simulink model "fixedWing"  (R2024b)
settings: Solver=ode1  StartTime=0.0  StopTime=20  FixedStep=0.001  RelTol=1e-3
undefined symbols (not defined in the file): initial_fw_state, params
libraries: uavutilslib x1
settings Model: PacingRate=0.010000  Creator=William Riis  LastModifiedBy=William Riis
settings DataIOCC: SaveFormat=StructureWithTime  SaveState=on

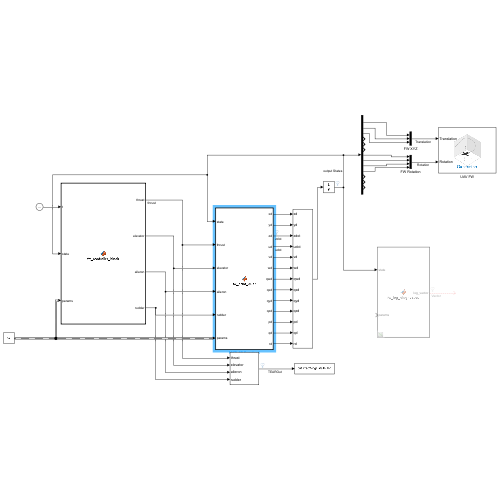
[thumbnail: Simulink's stored preview of the top-level diagram]
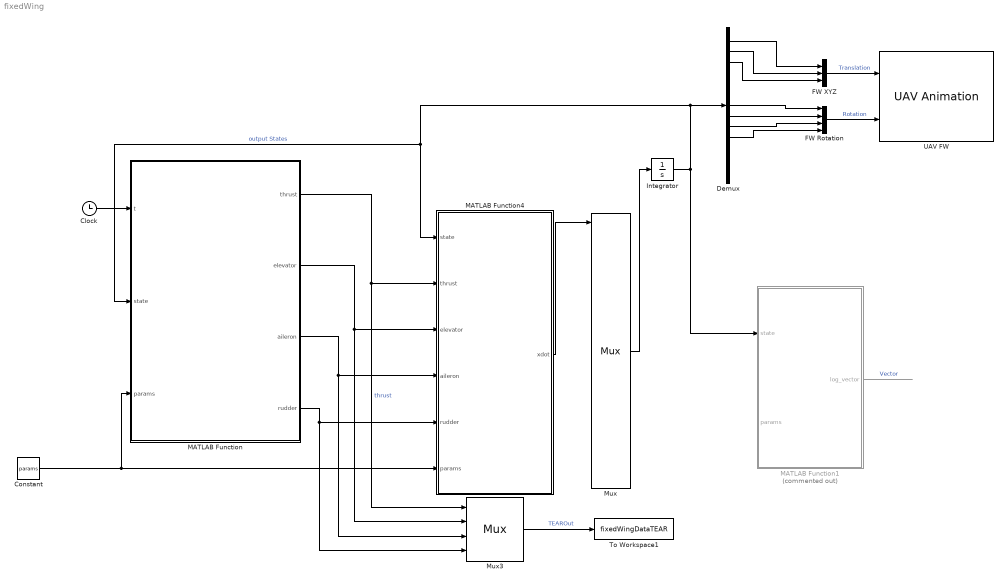
== system fixedWing ==
  Clock : Clock
  Constant : Constant  Value=params  OutDataTypeStr=Bus: paramsBus
  Demux : Demux  Outputs=13
  FW Rotation : Mux
  FW XYZ : Mux  Inputs=3
  Integrator : Integrator  InitialCondition=initial_fw_state
  MATLAB Function : MATLAB Function  TreatAsAtomicUnit=on
  MATLAB Function1 : MATLAB Function  Commented=on  TreatAsAtomicUnit=on
  MATLAB Function4 : MATLAB Function  TreatAsAtomicUnit=on
  Mux : Mux  Inputs=13
      settings: DisplayOption=signals
  Mux3 : Mux
      settings: DisplayOption=signals
  To Workspace1 : ToWorkspace  VariableName=fixedWingDataTEAR  SaveFormat=Structure With Time  SampleTime=-1
      settings: Save2DSignal=2-D array (concatenate along first dimension)
  UAV FW : uavutilslib/UAV Animation  NumUAV=1  DynamicUAVConfig=off  UAVType=FixedWing  UAVSize=20  UAVColor=[1 0 0]  UAVTrajectoryAlpha=1  InertialZDirection=Down  RotationFormat=Quaternion  DrawMarkers=off  SampleTime=.01
  wires:
  Integrator/1 -> MATLAB Function1/1(state), Demux/1, MATLAB Function4/1(state), MATLAB Function/2(state)  "output States"
  Mux3/1 -> To Workspace1/1  "TEAROut"
  FW XYZ/1 -> UAV FW/1  "Translation"
  MATLAB Function/4(rudder) -> Mux3/4, MATLAB Function4/5(rudder)
  MATLAB Function/3(aileron) -> Mux3/3, MATLAB Function4/4(aileron)
  MATLAB Function/2(elevator) -> Mux3/2, MATLAB Function4/3(elevator)
  MATLAB Function/1(thrust) -> Mux3/1, MATLAB Function4/2(thrust)  "thrust"
  FW Rotation/1 -> UAV FW/2  "Rotation"
  Mux/1 -> Integrator/1
  Clock/1 -> MATLAB Function/1(t)
  MATLAB Function1/1(log_vector) -> ?  "Vector"
  Demux/1 -> FW XYZ/1
  Demux/2 -> FW XYZ/2
  Demux/3 -> FW XYZ/3
  Demux/7 -> FW Rotation/1
  Demux/8 -> FW Rotation/2
  Demux/9 -> FW Rotation/3
  Demux/10 -> FW Rotation/4
  MATLAB Function4/1(xdot) -> Mux/1
  ? -> Mux/2
  ? -> Mux/3  "zdot"
  ? -> Mux/4  "udot"
  ? -> Mux/5
  ? -> Mux/6
  ? -> Mux/7
  ? -> Mux/8
  ? -> Mux/9
  ? -> Mux/10
  ? -> Mux/11
  ? -> Mux/12
  ? -> Mux/13
  Constant/1 -> MATLAB Function/3(params), MATLAB Function4/6(params)

== matlab function fixedWing/MATLAB Function1 ==
  data: state input; log_vector output; params input
function log_vector = fw_log_diagnostics(state, params)
% Logs diagnostics from aircraft state for debugging purposes

% === Unpack State ===
u = state(4); v = state(5); w = state(6);
phi = state(7); theta = state(8); psi = state(9);

% === Aircraft Constants (Fixed-Wing Specific with Prefixes) ===
rho = params.rho;
S   = params.fw_S;
CL0 = params.fw_CL0;
CL_alpha = params.fw_CL_alpha;
CD0 = params.fw_CD0;
k   = params.fw_k;

% === Velocity & Angles ===
V_b = [u; v; w];
V = norm(V_b) + 1e-3;
alpha = atan2(w, u);
qbar = 0.5 * rho * V^2;

% === Aero Coefficients & Forces ===
CL = CL0 + CL_alpha * alpha;
CD = CD0 + k * CL^2;
L = CL * qbar * S;
D = CD * qbar * S;

% === Direction Vectors ===
V_hat = V_b / V;
drag_dir = -V_hat;
lift_dir = cross([0; 1; 0], drag_dir);
lift_dir = lift_dir / max(1e-6, norm(lift_dir));

% === Logged Output Vector ===
% [V, alpha, CL, CD, L, D, V_hat(1:3), lift_dir(1:3)]
log_vector = [V; alpha; CL; CD; L; D; V_hat; lift_dir];
end

== matlab function fixedWing/MATLAB Function4 ==
  data: state input; thrust input; elevator input; aileron input; rudder input; xdot output; params input
function xdot = fw_6dof_quat(state, thrust, elevator, aileron, rudder, params)
% FW_6DOF_QUAT  Rigid-body 6-DoF fixed-wing with wind-axis aero
%
% State (13x1): [x y z u v w q0 q1 q2 q3 p q r]'
%   x,y,z   : position in NED (m)  (Z down)
%   u,v,w   : body translational velocities (m/s)  (inertial-relative)
%   q0..q3  : quaternion q_BN (N->Body), scalar-first (Hamilton)
%   p,q,r   : body rates (rad/s)
%
% Inputs:
%   thrust   : propulsive thrust along +x_B (N)
%   elevator : elevator deflection (rad)
%   aileron  : aileron deflection  (rad)
%   rudder   : rudder deflection   (rad)
%
% Params (required fields; uses safe defaults if missing):
%   rho,S,b,c,g, wind_ned(3x1)
%   Ix,Iy,Iz,Ixz (preferred) OR J (3x3)
%   Aero coeffs: CL0, CL_alpha, CL_q, CL_de,
%                CD0, k (=induced), CDa, CD_q, CD_de,
%                CY_beta, CY_p, CY_r, CY_da, CY_dr,
%                Cl_beta, Cl_p, Cl_r, Cl_da, Cl_dr,
%                Cm0, Cm_alpha, Cm_q, Cm_de,
%                Cn_beta, Cn_p, Cn_r, Cn_da, Cn_dr
%   r_T (3x1): thrust offset from CG in body (m), optional (default [0;0;0])

% -------- unpack state
x = state(1); y = state(2); z = state(3); %#ok<NASGU>
u = state(4); v = state(5); w = state(6);
qBN = state(7:10);
p = state(11); q = state(12); r = state(13);

% -------- params & defaults
rho  = getdef(params,'rho',1.225);
S    = getdef(params,'S',0.25);
b    = getdef(params,'b',1.2);
c    = getdef(params,'c',S/max(b,eps));
g    = getdef(params,'g',9.81);
wind = getdef(params,'wind_ned',[0;0;0]);

% Inertia (allow Ixz coupling)
if all(isfield(params, {'Ix','Iy','Iz'}))
    Ix  = params.Ix; Iy = params.Iy; Iz = params.Iz;
    Ixz = getdef(params,'Ixz',0);
    J   = [Ix, 0, -Ixz;
           0,  Iy, 0;
          -Ixz,0,  Iz];
else
    J = getdef(params,'J',diag([0.045 0.065 0.085]));
end

% Aero coefficients (provide zeros if missing)
CL0   = getdef(params,'CL0',0);
CL_a  = getdef(params,'CL_alpha',0);
CL_q  = getdef(params,'CL_q',0);
CL_de = getdef(params,'CL_de',0);

CD0   = getdef(params,'CD0',0.01);
k_ind = getdef(params,'k',0.03);
CD_a  = getdef(params,'CDa',0);
CD_q  = getdef(params,'CD_q',0);
CD_de = getdef(params,'CD_de',0);

CY_b  = getdef(params,'CY_beta',0);
CY_p  = getdef(params,'CY_p',0);
CY_r  = getdef(params,'CY_r',0);
CY_da = getdef(params,'CY_da',0);
CY_dr = getdef(params,'CY_dr',0);

Cl_b  = getdef(params,'Cl_beta',0);
Cl_p  = getdef(params,'Cl_p',0);
Cl_r  = getdef(params,'Cl_r',0);
Cl_da = getdef(params,'Cl_da',0);
Cl_dr = getdef(params,'Cl_dr',0);

Cm0   = getdef(params,'Cm0',0);
Cm_a  = getdef(params,'Cm_alpha',0);
Cm_q  = getdef(params,'Cm_q',0);
Cm_de = getdef(params,'Cm_de',0);

Cn_b  = getdef(params,'Cn_beta',0);
Cn_p  = getdef(params,'Cn_p',0);
Cn_r  = getdef(params,'Cn_r',0);
Cn_da = getdef(params,'Cn_da',0);
Cn_dr = getdef(params,'Cn_dr',0);

r_T = getdef(params,'r_T',[0;0;0]);

% -------- rotations
R_BN = quatNED_to_body(qBN);  % N->B
R_NB = R_BN.';                % B->N

% -------- kinematics: position time-derivative in NED
v_b   = [u; v; w];
v_ned = R_NB * v_b;
x_dot = v_ned(1);
y_dot = v_ned(2);
z_dot = v_ned(3);

% -------- air-relative velocity in body
v_air_b = v_b - R_BN*wind;    % (R_BN*wind) is wind expressed in body
ua = v_air_b(1); va = v_air_b(2); wa = v_air_b(3);
Va = max(1e-3, norm(v_air_b));

alpha = atan2(wa, ua);                     % angle of attack
beta  = asin( clamp(va/Va, -1, 1) );       % sideslip

qbar = 0.5 * rho * Va^2;
p_hat = (b/(2*Va)) * p;
q_hat = (c/(2*Va)) * q;
r_hat = (b/(2*Va)) * r;

% -------- aerodynamic coefficients
CL = CL0 + CL_a*alpha + CL_q*q_hat + CL_de*elevator;
CD = CD0 + k_ind*CL^2 + CD_a*alpha + CD_q*q_hat + CD_de*elevator;
CY = CY_b*beta + CY_p*p_hat + CY_r*r_hat + CY_da*aileron + CY_dr*rudder;

Cl = Cl_b*beta + Cl_p*p_hat + Cl_r*r_hat + Cl_da*aileron + Cl_dr*rudder;
Cm = Cm0 + Cm_a*alpha + Cm_q*q_hat + Cm_de*elevator;
Cn = Cn_b*beta + Cn_p*p_hat + Cn_r*r_hat + Cn_da*aileron + Cn_dr*rudder;

% -------- wind-axis → body conversion for forces
% In wind axes, F_w = [ -D,  Y,  -L ] * qbar*S
F_w = qbar*S * [-CD; CY; -CL];

% Rotation from body->wind (C_b^w), then use its transpose for wind->body
ca = cos(alpha); sa = sin(alpha);
cb = cos(beta);  sb = sin(beta);
C_b_w = [  ca*cb,  sb,    sa*cb;
          -ca*sb,  cb,   -sa*sb;
          -sa,     0,      ca  ];
R_wb = C_b_w.';               % wind -> body
F_aero_b = R_wb * F_w;

% -------- aerodynamic moments in body
M_aero_b = qbar*S * [ b*Cl; c*Cm; b*Cn ];

% -------- thrust force & moment
F_thrust_b = [thrust; 0; 0];
M_thrust_b = cross(r_T(:), F_thrust_b);

% -------- gravity in body
F_grav_b = R_BN * [0;0; g*getdef(params,'m',1.0)]; % using FW mass if provided
m_fw = getdef(params,'m',1.0);

% -------- total body forces & accelerations
F_b = F_aero_b + F_thrust_b + F_grav_b;

% body translational dynamics:  v̇_b = (1/m)F_b - ω×v_b
omega = [p;q;r];
v_dot_b = (1/m_fw) * F_b - cross(omega, v_b);

u_dot = v_dot_b(1);
v_dot = v_dot_b(2);
w_dot = v_dot_b(3);

% -------- attitude kinematics (quaternion)
Omega = [ 0   -p   -q   -r;
          p    0    r   -q;
          q   -r    0    p;
          r    q   -p    0 ];
q_dot = 0.5 * Omega * qBN;     % (normalize after integration in driver)

% -------- rotational dynamics
M_b = M_aero_b + M_thrust_b;
omega_dot = J \ ( M_b - cross(omega, J*omega) );
p_dot = omega_dot(1);
q_dotb = omega_dot(2);
r_dot = omega_dot(3);

% -------- assemble derivative
xdot = zeros(13,1);
xdot(1)  = x_dot;
xdot(2)  = y_dot;
xdot(3)  = z_dot;
xdot(4)  = u_dot;
xdot(5)  = v_dot;
xdot(6)  = w_dot;
xdot(7:10) = q_dot;
xdot(11) = p_dot;
xdot(12) = q_dotb;
xdot(13) = r_dot;

end

% ===================== helpers ==========================
function R = quatNED_to_body(q)
% q = [q0 q1 q2 q3] (scalar-first), mapping NED -> Body (Hamilton)
q0 = q(1); q1 = q(2); q2 = q(3); q3 = q(4);
R = [ 1-2*(q2^2+q3^2),   2*(q1*q2 + q0*q3),  2*(q1*q3 - q0*q2);
      2*(q1*q2 - q0*q3), 1-2*(q1^2+q3^2),    2*(q2*q3 + q0*q1);
      2*(q1*q3 + q0*q2), 2*(q2*q3 - q0*q1),  1-2*(q1^2+q2^2) ];
end

function y = clamp(x, a, b)
y = min(max(x,a), b);
end

function out = getdef(S, field, defaultVal)
if isfield(S, field), out = S.(field); else, out = defaultVal; end
end

== matlab function fixedWing/MATLAB Function ==
  settings: updateMethod=DISCRETE
  data: t input; thrust output; elevator output; aileron output; rudder output; state input; params input
function [thrust, elevator, aileron, rudder] = fw_controller_block(t, state, params)
% Scripted maneuver controller for dynamic model validation
% Inputs:
%   t      : simulation time [s]
%   state  : 13x1 state vector [x y z u v w q0 q1 q2 q3 p q r]
%   params : parameter struct (must include .min_thrust, .max_thrust)

% ==== Trim and Control Gains ====
target_speed   = 6.0;       % m/s
trim_thrust    = 3.5;       % N
trim_elevator  = -0.07;     % rad
K_thrust       = 0.5;

% ==== Damping Gains ====
Kp_aileron  = 0.3;
Kp_elevator = 0.3;
Kp_rudder   = 0.2;

% ==== Extract States ====
u = state(4); v = state(5); w = state(6);
p = state(11); q = state(12); r = state(13);

% ==== Airspeed ====
V = sqrt(u^2 + v^2 + w^2);

% ==== Base Trim Inputs ====
elevator_cmd = trim_elevator;
aileron_cmd  = 0.0;

% ==== Time-based Maneuver Sequence ====
% Each maneuver lasts ~2 seconds
if t >= 3 && t < 5
    aileron_cmd = 0.25;      % Bank right (~15°)
elseif t >= 5 && t < 7
    aileron_cmd = 0.0;       % Level out
elseif t >= 7 && t < 9
    aileron_cmd = -0.45;     % Stronger bank left (~25°)
elseif t >= 9 && t < 11
    aileron_cmd = 0.0;       % Level out
elseif t >= 11 && t < 13
    elevator_cmd = -0.25;    % Climb (pitch up ~10°)
elseif t >= 13 && t < 15
    elevator_cmd = trim_elevator;  % Level off
elseif t >= 15 && t < 17
    elevator_cmd = 0.10;     % Dive (pitch down ~-10°)
else
    elevator_cmd = trim_elevator;  % Final level flight
end

% ==== Thrust Control with Climb Boost ====
thrust = trim_thrust + K_thrust * (target_speed - V);

if t >= 11 && t < 13
    thrust = thrust + 1.0;   % Boost during climb
end

% Saturate thrust
thrust = min(max(thrust, params.min_thrust), params.max_thrust);

% ==== Control Outputs with Rate Damping ====
aileron  = aileron_cmd - Kp_aileron  * p;
elevator = elevator_cmd - Kp_elevator * q;
rudder   = -Kp_rudder * r;
end
